simulink model "connection5_first"  (R2017b)
settings: Solver=VariableStepAuto  StartTime=0.0  StopTime=50  RelTol=1e-3
values from neighbouring files (symbols this model uses):
  A5 = [-2,0,0,0,0,0,0,0,1,0 ... (first row only)    [param.m]
  D1_5 = [(d1(1,1)-d1(5,1))+d1(1,1) ... (first row only)    [param.m]
  K1 = 1    [param.m]
  start = [0;1.5;0;-1.5;-3;3;-3;0;-3;-3]    [param.m]
settings Model: Creator=yunfei  LastModifiedBy=yunfei

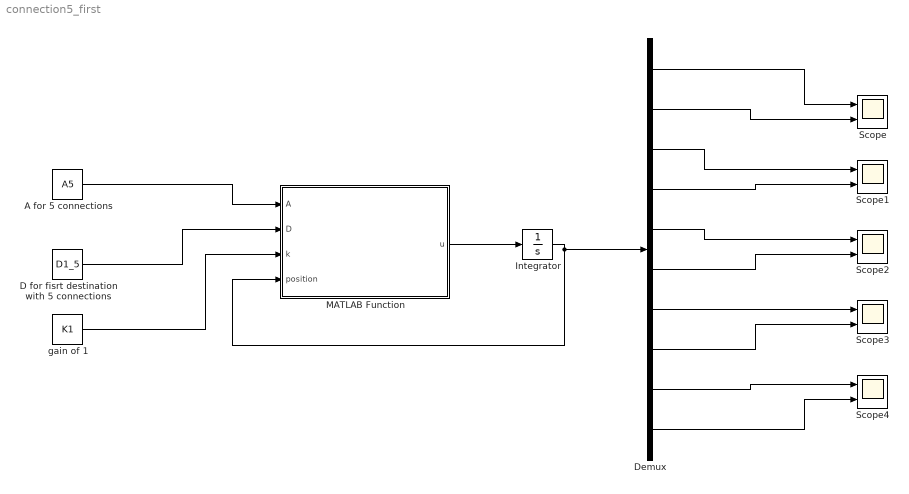
== system connection5_first ==
  A for 5 connections : Constant  Value=A5
  "D for fisrt destination with 5 connections " : Constant  Value=D1_5
  Demux : Demux  Outputs=10
  Integrator : Integrator  InitialCondition=start
  MATLAB Function : MATLAB Function  TreatAsAtomicUnit=on
  Scope{,1..4} (5 alike) : Scope  NumInputPorts=2
  gain of 1 : Constant  Value=K1
  wires:
  A for 5 connections/1 -> MATLAB Function/1(A)
  "D for fisrt destination with 5 connections "/1 -> MATLAB Function/2(D)
  gain of 1/1 -> MATLAB Function/3(k)
  MATLAB Function/1(u) -> Integrator/1
  Integrator/1 -> MATLAB Function/4(position), Demux/1
  Demux/1 -> Scope/1
  Demux/2 -> Scope/2
  Demux/3 -> Scope1/1
  Demux/4 -> Scope1/2
  Demux/5 -> Scope2/1
  Demux/6 -> Scope2/2
  Demux/7 -> Scope3/1
  Demux/8 -> Scope3/2
  Demux/9 -> Scope4/1
  Demux/10 -> Scope4/2

== matlab function connection5_first/MATLAB Function ==
  data: A input; u output; D input; k input; position input
function u = fcn(A, D, k, position)
    u = k.*A * position + D;
end
